simulink library "dlbsBlockParameterUpdate"  (R2025b)
settings: Solver=VariableStepAuto  StartTime=0.0  StopTime=10.0  RelTol=1e-3
libraries: dlbsBlockInsertGradientGF x1
settings Model: Creator=lt6037  LastModifiedBy=lt6037

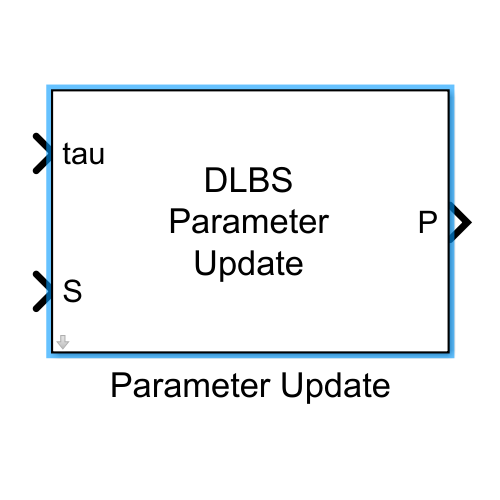
[thumbnail: Simulink's stored preview of the top-level diagram]
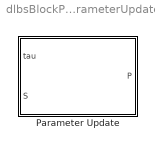
== system dlbsBlockParameterUpdate ==
  Parameter Update : Subsystem
      mask help: Updates an parameter P state using a source tensor S and mixing factor tau.
      mask Help: web("dlbsHelpBlockParameterUpdate.html")
      mask Display: fprintf("DLBS\nParameter\nUpdate")

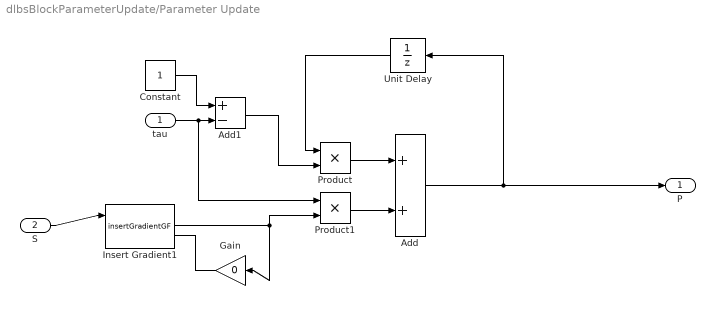
== system dlbsBlockParameterUpdate/Parameter Update ==
  tau : Inport
  S : Inport  Port=2
  Add : Sum
  Add1 : Sum  Inputs=+-
  Constant : Constant
  Gain : Gain  Gain=0
  Insert Gradient1 : dlbsBlockInsertGradientGF/insertGradientGF
  Product : Product
  Product1 : Product
  Unit Delay : UnitDelay  SampleTime=-1  HasFrameUpgradeWarning=on
  P : Outport
  wires:
  Product/1 -> Add/1
  Unit Delay/1 -> Product/1
  Constant/1 -> Add1/1
  Add1/1 -> Product/2
  Product1/1 -> Add/2
  tau/1 -> Product1/1, Add1/2
  Insert Gradient1/1 -> Gain/1, Product1/2
  Add/1 -> P/1, Unit Delay/1
  S/1 -> Insert Gradient1/1
  Gain/1 -> Insert Gradient1/2
